simulink model "control_effort"  (R2019b)
settings: Solver=VariableStepAuto  StartTime=0.0  StopTime=20.0  RelTol=1e-3
libraries: simulink x1
settings Model: Creator=mmd  LastModifiedBy=mmd

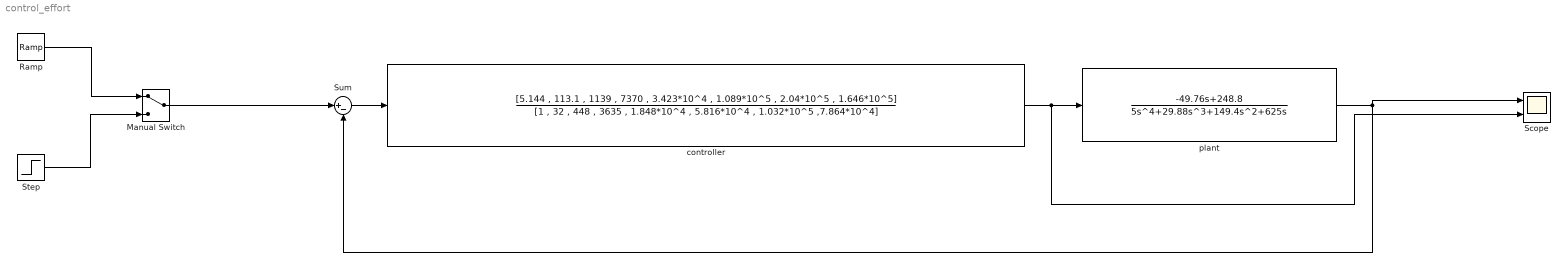
== system control_effort ==
  Manual Switch : ManualSwitch
  Ramp : simulink/Sources/Ramp  slope=1  start=0  InitialOutput=0
  Scope : Scope  NumInputPorts=2
  Step : Step  SampleTime=0
  Sum : Sum  Inputs=|+-
  controller : TransferFcn  Numerator=[5.144 , 113.1 , 1139 , 7370 , 3.423*10^4 , 1.089*10^5 , 2.04*10^5 , 1.646*10^5]  Denominator=[1 , 32 , 448 , 3635 , 1.848*10^4 , 5.816*10^4 , 1.032*10^5 ,7.864*10^4]
  "plant " : TransferFcn  Numerator=[-49.76,248.8]  Denominator=[5 ,29.88 ,149.4 ,625 ,0 ]
  wires:
  Ramp/1 -> Manual Switch/1
  Step/1 -> Manual Switch/2
  Manual Switch/1 -> Sum/1
  Sum/1 -> controller/1
  controller/1 -> "plant "/1, Scope/2
  "plant "/1 -> Scope/1, Sum/2
